simulink model "BasePerTracing_ESTIM"  (R2023a)
settings: Solver=FixedStepDiscrete  StartTime=0.0  StopTime=Inf  RelTol=1e-3  EnableMultiTasking=on
InitFcn:
  | mcb_pmsm_foc_qep_f28379d_data;
values from neighbouring files (symbols this model uses):
  ADCCount = ADCResolution-1    (= 4095)    [BaseModelForControl_Parameters_DAHLIN.m]    (also in BaseModelForControl_Parameters_DEADBEAT.m; BaseModelForControl_Parameters_ESTIM.m; BaseModelForControl_Parameters_PI.m)
  GainVsense = 4.99/(62+4.99)    (= 0.0744887296611)    [BaseModelForControl_Parameters_DAHLIN.m]    (also in BaseModelForControl_Parameters_DEADBEAT.m; BaseModelForControl_Parameters_ESTIM.m; BaseModelForControl_Parameters_PI.m)
  J = Jdc+Jbr    (= 7.32e-05)    [BaseModelForControl_Parameters_DAHLIN.m]    (also in BaseModelForControl_Parameters_DEADBEAT.m; BaseModelForControl_Parameters_ESTIM.m; BaseModelForControl_Parameters_PI.m; DAHLINModel_Parameters.m = 8.3561e-05)
  km = 0.12    [BaseModelForControl_Parameters_DAHLIN.m]    (also in BaseModelForControl_Parameters_DEADBEAT.m; BaseModelForControl_Parameters_ESTIM.m; BaseModelForControl_Parameters_PI.m; DAHLINModel_Parameters.m)
  KpI = La_estim/taui    (= 6.1)    [BaseModelForControl_Parameters_DAHLIN.m]    (also in BaseModelForControl_Parameters_DEADBEAT.m; BaseModelForControl_Parameters_ESTIM.m; BaseModelForControl_Parameters_PI.m)
  KpW = J_estim/(tauw*km)    (= 0.0696341666667)    [BaseModelForControl_Parameters_DAHLIN.m]    (also in BaseModelForControl_Parameters_DEADBEAT.m; BaseModelForControl_Parameters_ESTIM.m; BaseModelForControl_Parameters_PI.m)
  OffsetADCINC4 = 2284    [BaseModelForControl_Parameters_DAHLIN.m]    (also in BaseModelForControl_Parameters_DEADBEAT.m; BaseModelForControl_Parameters_ESTIM.m; BaseModelForControl_Parameters_PI.m)
  PulseNumber = 2048*4    (= 8192)    [BaseModelForControl_Parameters_DAHLIN.m]    (also in BaseModelForControl_Parameters_DEADBEAT.m; BaseModelForControl_Parameters_ESTIM.m; BaseModelForControl_Parameters_PI.m; DAHLINModel_Parameters.m)
  RadiantsPerCount = 2*pi/(PulseNumber-1)    (= 0.00076708403213)    [BaseModelForControl_Parameters_DAHLIN.m]    (also in BaseModelForControl_Parameters_DEADBEAT.m; BaseModelForControl_Parameters_ESTIM.m; BaseModelForControl_Parameters_PI.m; DAHLINModel_Parameters.m)
  RpmToRads = 2*pi/60    (= 0.10471975512)    [BaseModelForControl_Parameters_DAHLIN.m]    (also in BaseModelForControl_Parameters_DEADBEAT.m; BaseModelForControl_Parameters_ESTIM.m; BaseModelForControl_Parameters_PI.m; DAHLINModel_Parameters.m)
  TaoFilterOffsetCurrent = 1    [BaseModelForControl_Parameters_DAHLIN.m]    (also in BaseModelForControl_Parameters_DEADBEAT.m; BaseModelForControl_Parameters_ESTIM.m; BaseModelForControl_Parameters_PI.m)
  TaoFilterOmega = 0.001    [BaseModelForControl_Parameters_DAHLIN.m]    (also in BaseModelForControl_Parameters_DEADBEAT.m; BaseModelForControl_Parameters_ESTIM.m; BaseModelForControl_Parameters_PI.m; DAHLINModel_Parameters.m)
  TiI = tauel_new    (= 0.00182804399293)    [BaseModelForControl_Parameters_DAHLIN.m]    (also in BaseModelForControl_Parameters_DEADBEAT.m; BaseModelForControl_Parameters_ESTIM.m; BaseModelForControl_Parameters_PI.m)
  TiW = taumecc_new    (= 0.0974313231659)    [BaseModelForControl_Parameters_DAHLIN.m]    (also in BaseModelForControl_Parameters_DEADBEAT.m; BaseModelForControl_Parameters_ESTIM.m; BaseModelForControl_Parameters_PI.m)
  TSample = PWM_Period    (= 0.0001)    [BaseModelForControl_Parameters_DAHLIN.m]    (also in BaseModelForControl_Parameters_DEADBEAT.m; BaseModelForControl_Parameters_ESTIM.m; BaseModelForControl_Parameters_PI.m; DAHLINModel_Parameters.m)
  VrefADC = 3    [BaseModelForControl_Parameters_DAHLIN.m]    (also in BaseModelForControl_Parameters_DEADBEAT.m; BaseModelForControl_Parameters_ESTIM.m; BaseModelForControl_Parameters_PI.m)
undefined symbols (not defined in the file or in its folder): dataType, Down, GPTRIP1SEL, GPTRIP2SEL, TZ1, TZ2, Up
libraries: c2802xlib x9, simulink x9, c2837xDlib x4, c280xlib x4, c2000lib x1, svdutilitieslib x1
(part 2 of 2)

== system BasePerTracing_ESTIM/Serial Receive/Data_Conditioning_Rx/Data_Type_Fixed_Point ==
  In1 : Inport
  Data Type Conversion1 : DataTypeConversion  OutDataTypeStr=dataType  RndMeth=Simplest  SaturateOnIntegerOverflow=off
  Data Type Conversion2 : DataTypeConversion  OutDataTypeStr=fixdt(1,32,28)  ConvertRealWorld=Stored Integer (SI)  RndMeth=Simplest  SaturateOnIntegerOverflow=off
  Data Type Conversion3 : DataTypeConversion  OutDataTypeStr=uint16  RndMeth=Simplest  SaturateOnIntegerOverflow=off
  Demux : Demux  Outputs=2
  Desired Speed : Outport
  Out2 : Outport  Port=2
  wires:
  In1/1 -> Demux/1
  Data Type Conversion1/1 -> Desired Speed/1
  Data Type Conversion2/1 -> Data Type Conversion1/1
  Demux/1 -> Data Type Conversion2/1
  Demux/2 -> Data Type Conversion3/1
  Data Type Conversion3/1 -> Out2/1

== system BasePerTracing_ESTIM/Serial Receive/Data_Conditioning_Rx/Data_Type_Float ==
  In1 : Inport
  Data Type Conversion2 : DataTypeConversion  OutDataTypeStr=uint16  RndMeth=Simplest  SaturateOnIntegerOverflow=off
  Demux : Demux  Outputs=2
  Desired Speed : Outport
  Out2 : Outport  Port=2
  wires:
  In1/1 -> Demux/1
  Demux/1 -> Desired Speed/1
  Data Type Conversion2/1 -> Out2/1
  Demux/2 -> Data Type Conversion2/1

== system BasePerTracing_ESTIM/Current Control/SCI (Code Generation)/Data_Conditioning_Tx/Data_Type_Fixed_Point ==
  In1 : Inport
  Data Type Conversion : DataTypeConversion  OutDataTypeStr=fixdt(1,32,28)  RndMeth=Simplest  SaturateOnIntegerOverflow=off
  Data Type Conversion3 : DataTypeConversion  OutDataTypeStr=uint32  ConvertRealWorld=Stored Integer (SI)  RndMeth=Simplest  SaturateOnIntegerOverflow=off
  Data_Log : Outport
  wires:
  In1/1 -> Data Type Conversion/1
  Data Type Conversion3/1 -> Data_Log/1
  Data Type Conversion/1 -> Data Type Conversion3/1

== system BasePerTracing_ESTIM/Current Control/SCI (Code Generation)/Data_Conditioning_Tx/Data_Type_Float ==
  In1 : Inport
  Byte Pack : svdutilitieslib/Byte Pack  maskPackedDataType=uint32  datatypes={'single'}  byteAlign=4  blockPlatform=tic2000
  Data_Log : Outport
  wires:
  Byte Pack/1 -> Data_Log/1
  In1/1 -> Byte Pack/1

== system BasePerTracing_ESTIM/Current Control/SCI (Code Generation)/Data_Logging/Data ==
  Data : Inport
  Data_width : Inport  Port=2
  Action Port : ActionPort  ActionPortLabel=else
  Dummy : Constant  Value=hex2dec('0000')  OutDataTypeStr=uint32
  Mux : Mux  Inputs=2
  Data_out : Outport  VectorParamsAs1DForOutWhenUnconnected=off
  Iteration : Outport  Port=2  VectorParamsAs1DForOutWhenUnconnected=off
  wires:
  Data_width/1 -> Iteration/1
  Data/1 -> Mux/1
  Dummy/1 -> Mux/2
  Mux/1 -> Data_out/1

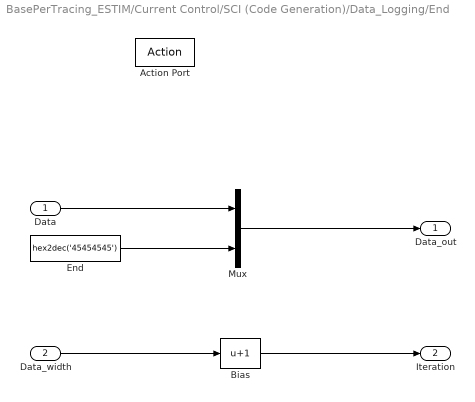
== system BasePerTracing_ESTIM/Current Control/SCI (Code Generation)/Data_Logging/End ==
  Data : Inport
  Data_width : Inport  Port=2
  Action Port : ActionPort  ActionPortLabel=elseif(u1 == 599)
  Bias : Bias  Bias=1  SaturateOnIntegerOverflow=off
  End : Constant  Value=hex2dec('45454545')  OutDataTypeStr=uint32
  Mux : Mux  Inputs=2
  Data_out : Outport  VectorParamsAs1DForOutWhenUnconnected=off
  Iteration : Outport  Port=2  VectorParamsAs1DForOutWhenUnconnected=off
  wires:
  Data/1 -> Mux/1
  Data_width/1 -> Bias/1
  Bias/1 -> Iteration/1
  End/1 -> Mux/2
  Mux/1 -> Data_out/1

== system BasePerTracing_ESTIM/Current Control/SCI (Code Generation)/Data_Logging/Start ==
  Data : Inport
  Data_width : Inport  Port=2
  Action Port : ActionPort  ActionPortLabel=if(u1 == 0)
  Bias : Bias  Bias=1  SaturateOnIntegerOverflow=off
  Mux : Mux  Inputs=2
  Start : Constant  Value=hex2dec('53535353')  OutDataTypeStr=uint32
  Data_out : Outport  VectorParamsAs1DForOutWhenUnconnected=off
  Iteration : Outport  Port=2  VectorParamsAs1DForOutWhenUnconnected=off
  wires:
  Data/1 -> Mux/2
  Data_width/1 -> Bias/1
  Bias/1 -> Iteration/1
  Start/1 -> Mux/1
  Mux/1 -> Data_out/1

== matlab function BasePerTracing_ESTIM/Current Control/AnalogReading/MATLAB Function ==
  data: Ts input; out output; Tao input; In input
function out  = LowPassFilter(  Ts ,Tao, In)

persistent OutPrecedente
if isempty( OutPrecedente )
    OutPrecedente = 0 ;
end
    %Filtro passa basso discretizzato con il metodo delle differenze
    %all'indietro
    
    a=Ts/(Ts+Tao);
    b=Tao/(Ts+Tao);
    
    out=a*In+OutPrecedente*b;
   
    OutPrecedente = out;
   
end

== matlab function BasePerTracing_ESTIM/Current Control/ENCODER/MATLAB Function1 ==
  data: Ts input; ThetaMis output; RadiantiPerCount input; Counter input; OmegaMis output; OmegaMisRPM output; DeltaCounter output
function [ThetaMis, OmegaMis, OmegaMisRPM, DeltaCounter] = CounterToThetaOmega(Ts, RadiantiPerCount, Counter)

% Inizializzazione dei valori iniziali 
persistent CounterPrec  
if isempty( CounterPrec )
    CounterPrec = 0;
end 

    DeltaCounter=Counter-CounterPrec;
    
    if (DeltaCounter>double(0x1000))
        DeltaCounter=DeltaCounter-double(0x2000);
    end
    
    if (DeltaCounter<-double(0x1000))
        DeltaCounter=DeltaCounter+double(0x2000);
    end
        
    % conversione conteggio in radianti
    ThetaMis = Counter * RadiantiPerCount;
    
    DeltaThetaMis = DeltaCounter*RadiantiPerCount;
   
    OmegaMis = DeltaThetaMis/Ts;
    OmegaMisRPM=OmegaMis*60/(2*pi);
 
    CounterPrec= Counter;
end

== matlab function BasePerTracing_ESTIM/Current Control/ENCODER/MATLAB Function ==
  data: Ts input; out output; Tao input; In input
function out  = LowPassFilter(  Ts ,Tao, In)

persistent OutPrecedente
if isempty( OutPrecedente )
    OutPrecedente = 0 ;
end
    %Filtro passa basso discretizzato con il metodo delle differenze
    %all'indietro
    
    a=Ts/(Ts+Tao);
    b=Tao/(Ts+Tao);
    
    out=a*In+OutPrecedente*b;
   
    OutPrecedente = out;
   
end

== matlab function BasePerTracing_ESTIM/Current Control/Subsystem/PI Current ==
  data: in input; out output; Kp input; Ti input; Ts input; Enable input; HighSat input; LowSat input; EnableCheckSat input
function out = PI(in, Kp, Ti, Ts, Enable, HighSat, LowSat, EnableCheckSat)
persistent in_prec out_prec

if isempty(out_prec)
    out_prec=0;
end

if isempty(in_prec)
    in_prec=0;
end
%G(s)=(Kp/Ti)*((1+Ti*s)/s) (Tustin)
% We run control only if motor is running
if(Enable==1)
     %I Calculate the output
     out = Kp*Ts/(2*Ti)*(in+in_prec) + Kp*(in-in_prec) + out_prec;
    if(EnableCheckSat == 1)

    %check for saturation
        if out > HighSat
            out = HighSat;
            % I calculate the input that gives me the saturated output
            in=(out-Kp*Ts/(2*Ti)*in_prec + Kp*in_prec - out_prec)/(Kp*Ts/(2*Ti)+Kp);
        elseif (out < LowSat)
            out = LowSat;
            in=(out-Kp*Ts/(2*Ti)*in_prec + Kp*in_prec - out_prec)/(Kp*Ts/(2*Ti)+Kp);
        end
     end
else
    out=0;
    in=0;
end
out_prec  = out;
in_prec=   in;
end

== matlab function BasePerTracing_ESTIM/Current Control/PI Current ==
  data: in input; out output; Kp input; Ti input; Ts input; Enable input; HighSat input; LowSat input; EnableCheckSat input; EnableAW input
function out = PI(in, Kp, Ti, Ts, Enable, HighSat, LowSat, EnableCheckSat, EnableAW)
persistent in_prec out_prec

if isempty(out_prec)
    out_prec=0;
end

if isempty(in_prec)
    in_prec=0;
end
%G(s)=(Kp/Ti)*((1+Ti*s)/s) (Tustin)
% We run control only if motor is running
if(Enable==1)
     %I Calculate the output
     out = Kp*Ts/(2*Ti)*(in+in_prec) + Kp*(in-in_prec) + out_prec;
    if(EnableCheckSat == 1)

    %check for saturation
        if out > HighSat
            out = HighSat;
            if (EnableAW==1)
                % I calculate the input that gives me the saturated output
                in=(out-Kp*Ts/(2*Ti)*in_prec + Kp*in_prec - out_prec)/(Kp*Ts/(2*Ti)+Kp); % AWUP
            end
        elseif (out < LowSat)
            out = LowSat;
            if(EnableAW==1)
                in=(out-Kp*Ts/(2*Ti)*in_prec + Kp*in_prec - out_prec)/(Kp*Ts/(2*Ti)+Kp); % AWUP
            end
        end
     end
else
    out=0;
    in=0;
end
out_prec  = out;
in_prec=   in;
end

== matlab function BasePerTracing_ESTIM/Current Control/Subsystem/PI Speed ==
  data: in input; out output; Kp input; Ti input; Ts input; Enable input; HighSat input; LowSat input; EnableCheckSat input
function out = PI(in, Kp, Ti, Ts, Enable, HighSat, LowSat, EnableCheckSat)
persistent in_prec out_prec

if isempty(out_prec)
    out_prec=0;
end

if isempty(in_prec)
    in_prec=0;
end
%G(s)=(Kp/Ti)*((1+Ti*s)/s) (Tustin)
% We run control only if motor is running
if(Enable==1)
     %I Calculate the output
     out = Kp*Ts/(2*Ti)*(in+in_prec) + Kp*(in-in_prec) + out_prec;
    if(EnableCheckSat == 1)

    %check for saturation
        if out > HighSat
            out = HighSat;
            % I calculate the input that gives me the saturated output
            in=(out-Kp*Ts/(2*Ti)*in_prec + Kp*in_prec - out_prec)/(Kp*Ts/(2*Ti)+Kp);
        elseif (out < LowSat)
            out = LowSat;
            in=(out-Kp*Ts/(2*Ti)*in_prec + Kp*in_prec - out_prec)/(Kp*Ts/(2*Ti)+Kp);
        end
     end
else
    out=0;
    in=0;
end
out_prec  = out;
in_prec=   in;
end

== matlab function BasePerTracing_ESTIM/Current Control/PI Speed ==
  data: in input; out output; Kp input; Ti input; Ts input; Enable input; HighSat input; LowSat input; EnableCheckSat input; EnableAW input
function out = PI(in, Kp, Ti, Ts, Enable, HighSat, LowSat, EnableCheckSat, EnableAW)
persistent in_prec out_prec

if isempty(out_prec)
    out_prec=0;
end

if isempty(in_prec)
    in_prec=0;
end
%G(s)=(Kp/Ti)*((1+Ti*s)/s) (Tustin)
% We run control only if motor is running
if(Enable==1)
     %I Calculate the output
     out = Kp*Ts/(2*Ti)*(in+in_prec) + Kp*(in-in_prec) + out_prec;
    if(EnableCheckSat == 1)

    %check for saturation
        if out > HighSat
            out = HighSat;
            if (EnableAW==1)
            % I calculate the input that gives me the saturated output
                in=(out-Kp*Ts/(2*Ti)*in_prec + Kp*in_prec - out_prec)/(Kp*Ts/(2*Ti)+Kp);
            end
        elseif (out < LowSat)
            out = LowSat;
            if (EnableAW == 1)
                in=(out-Kp*Ts/(2*Ti)*in_prec + Kp*in_prec - out_prec)/(Kp*Ts/(2*Ti)+Kp);
            end
        end
     end
else
    out=0;
    in=0;
end
out_prec  = out;
in_prec=   in;
end
